simulink model "MyPCImages"  (Simulink 7.5)
settings: Solver=FixedStepDiscrete  StartTime=0.0  StopTime=d_data(end,1)  FixedStep=apSampleTime  RelTol=1e-3
InitFcn:
  | replayFlight
values from neighbouring files (symbols this model uses):
  apSampleTime = 0.01    [demoz2SlugsV5.m]
  D = y    [BarOrthog.m]
  R0 = single(Euler2DCMdeg( PHI_IC, THETA_IC, PSI_IC ))    [demoz2SlugsV5.m]
undefined symbols (not defined in the file or in its folder): accBiasRateLimit, accelXCutTemp, axTGain1, axTGain2, axTMean1, axTMean2, barAdjust, baroCutoff, baroCutTemp, baroOffset, baroScale, barTGain1, barTGain2, barTMean1, barTMean2, baseHeight, baseTemp, cubeAccelGain, cubeGyroGain, gaind, GS_location, gyroBiasRateLimit, Init_onlyOnce, Init_Reset, ISA_rho0, lapseRate, lowRateSensorCutoff, magMeanTemp, magOffset, magScale, magTempK, mainSensorCutoff, maxDynPressure, param_acc, param_mag, pitAdjust, pitCutTemp, pitotOffset, pitotScale, pitTGain1, pitTGain2, pitTMean1, pitTMean2, polesd, powerOffset, powerScale, pressureSensorCutoff, T, tempOffset, tempScale, vzCutoff, xCutoff, yCutoff, zCutoff, zerosd
libraries: simulink x11, aerolibconvert2 x9, SLUGS_Library x6, aerolibutil x3, dspmtrx3 x3, dsPICdrivers x1
(part 1 of 4)
Description:
  | Rodrigues' formula for rotations, eq'n (12) of
  | Park, Chung, 'Geometric Integration on Euclidean
  | Group with Application to Articulated Multibody Systems', 2005
settings Model: Creator=Administrator  LastModifiedBy=Robert
settings OptimizationCC: InitFltsAndDblsToZero=on
settings DebuggingCC: SaveWithParameterizedLinksMsg=none  StrictBusMsg=Warning
settings GRTTargetCC: TargetFcnLib=ansi_tfl_tmw.mat

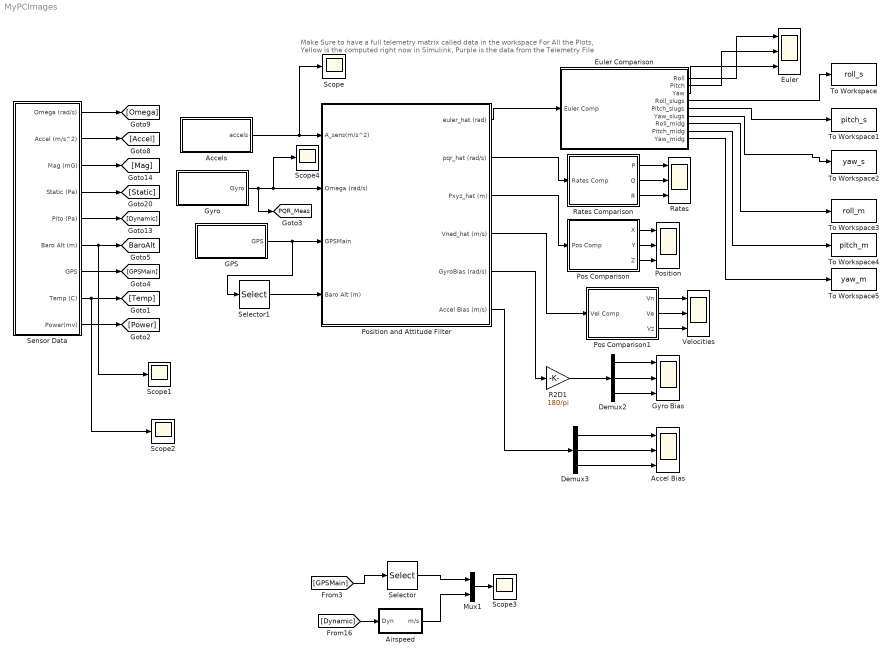
== system MyPCImages ==
  note: Make Sure to have a full telemetry matrix
      | called data in the workspace
      |
      | For All the Plots, Yellow is the computed right now in Simulink,
      |  Purple is the data from the Telemetry File
  Accel Bias : Scope  NumInputPorts=3
      settings: YMin=-0.05~-0.001~-1.73472e-018  YMax=0~0.0065~0.055  SaveName=ScopeData5
  Accels : Subsystem
  Airspeed : Subsystem
  Demux2 : Demux  Outputs=3
  Demux3 : Demux  Outputs=3
  Euler : Scope  NumInputPorts=3
      settings: YMin=-35~-7.5~0  YMax=10~10~400  SaveName=ScopeData15
  Euler Comparison : Subsystem
  GPS : Subsystem
  Gyro : Subsystem
  Gyro Bias : Scope  NumInputPorts=3
      settings: YMin=-0.1~5.55112e-017~-1  YMax=1~1.3~0.75  SaveName=ScopeData4
  Mux1 : Mux  Inputs=2
  Pos Comparison : Subsystem
  Pos Comparison1 : Subsystem
  Position : Scope  NumInputPorts=3
      settings: YMin=0~0~0  YMax=1.3e+006~2.25e+006~550000  SaveName=ScopeData2
  Position and Attitude Filter : Subsystem
  R2D1 : Gain  Gain=180/pi  ParameterDataType=sfix(16)  ParameterScaling=2^0  OutDataType=sfix(16)  OutScaling=2^0
  Rates : Scope  NumInputPorts=3
      settings: YMin=-150~-40~-70  YMax=150~80~40
  Rates Comparison : Subsystem
  Scope{,1..4} (5 alike) : Scope
      Scope settings: YMin=-22.5  YMax=15  SaveName=ScopeData10
      Scope1 settings: YMin=180  YMax=330  SaveName=ScopeData11
      Scope2 settings: TimeRange=300  YMin=-1200  YMax=400  SaveName=ScopeData6
      Scope3 settings: YMin=0  YMax=22.5  SaveName=ScopeData7
      Scope4 settings: YMin=-22.5  YMax=15
  Selector : Selector  InputPortWidth=5  IndexOptions=Index vector (dialog)  Indices=5  OutputSizes=1
  Selector1 : Selector  InputPortWidth=5  IndexOptions=Index vector (dialog)  Indices=3  OutputSizes=1
  Sensor Data : Subsystem
  To Workspace : ToWorkspace  VariableName=roll_s  SampleTime=-1  SaveFormat=Structure
  To Workspace1 : ToWorkspace  VariableName=pitch_s  SampleTime=-1  SaveFormat=Structure
  To Workspace2 : ToWorkspace  VariableName=yaw_s  SampleTime=-1  SaveFormat=Structure
  To Workspace3 : ToWorkspace  VariableName=roll_m  SampleTime=-1  SaveFormat=Structure
  To Workspace4 : ToWorkspace  VariableName=pitch_m  SampleTime=-1  SaveFormat=Structure
  To Workspace5 : ToWorkspace  VariableName=yaw_m  SampleTime=-1  SaveFormat=Structure
  Velocities : Scope  NumInputPorts=3
      settings: YMin=-25~-20~-15  YMax=25~25~17.5  SaveName=ScopeData3
  tag scope: BaroAlt=global, PQR_Meas=global
  wires:
  Accels/1(accels) -> Scope/1, Position and Attitude Filter/1(A_sens(m/s^2))
  GPS/1(GPS) -> Position and Attitude Filter/3(GPSMain), Selector1/1
  Sensor Data/2(Accel (m/s^2)) -> [Accel]
  Sensor Data/1(Omega (rad/s)) -> [Omega]
  Sensor Data/3(Mag (mG)) -> [Mag]
  Sensor Data/4(Static (Pa)) -> [Static]
  Sensor Data/5(Pito (Pa)) -> [Dynamic]
  Sensor Data/6(Baro Alt (m)) -> [BaroAlt], Scope1/1
  Sensor Data/7(GPS) -> [GPSMain]
  Sensor Data/8(Temp (C)) -> [Temp], Scope2/1
  Sensor Data/9(Power(mv)) -> [Power]
  Position and Attitude Filter/1(euler_hat (rad)) -> Euler Comparison/1(Euler Comp)
  Rates Comparison/1(P) -> Rates/1
  Rates Comparison/2(Q) -> Rates/2
  Rates Comparison/3(R) -> Rates/3
  Pos Comparison/3(Z) -> Position/3
  Position and Attitude Filter/3(Pxyz_hat (m)) -> Pos Comparison/1(Pos Comp)
  Pos Comparison/1(X) -> Position/1
  Pos Comparison/2(Y) -> Position/2
  Position and Attitude Filter/4(Vned_hat (m/s)) -> Pos Comparison1/1(Vel Comp)
  Demux2/3 -> Gyro Bias/3
  Demux2/2 -> Gyro Bias/2
  Demux2/1 -> Gyro Bias/1
  Position and Attitude Filter/5(GyroBias (rad/s)) -> R2D1/1
  Demux3/3 -> Accel Bias/3
  Demux3/2 -> Accel Bias/2
  Position and Attitude Filter/6(Accel Bias (m/s)) -> Demux3/1
  Demux3/1 -> Accel Bias/1
  Position and Attitude Filter/2(pqr_hat (rad/s)) -> Rates Comparison/1(Rates Comp)
  Pos Comparison1/1(Vn) -> Velocities/1
  Pos Comparison1/2(Ve) -> Velocities/2
  Pos Comparison1/3(Vz) -> Velocities/3
  R2D1/1 -> Demux2/1
  Gyro/1(Gyro) -> Position and Attitude Filter/2(Omega (rad/s)), Scope4/1, [PQR_Meas]
  Selector1/1 -> Position and Attitude Filter/4(Baro Alt (m))
  [Dynamic] -> Airspeed/1(Dyn)
  [GPSMain] -> Selector/1
  Selector/1 -> Mux1/1
  Airspeed/1(m/s) -> Mux1/2
  Mux1/1 -> Scope3/1
  Euler Comparison/1(Roll) -> Euler/1
  Euler Comparison/2(Pitch) -> Euler/2
  Euler Comparison/3(Yaw) -> Euler/3
  Euler Comparison/4(Roll_slugs) -> To Workspace/1
  Euler Comparison/5(Pitch_slugs) -> To Workspace1/1
  Euler Comparison/6(Yaw_slugs) -> To Workspace2/1
  Euler Comparison/7(Roll_midg) -> To Workspace3/1
  Euler Comparison/8(Pitch_midg) -> To Workspace4/1
  Euler Comparison/9(Yaw_midg) -> To Workspace5/1

== system MyPCImages/Accels ==
  Data Type Conversion : DataTypeConversion  OutDataTypeMode=single  OutDataType=sfix(16)  OutScaling=2^0  OutDataTypeStr=single
  Mux : Mux  Inputs=3
  p : FromWorkspace  VariableName=[d_data(:,1) d_data(:,5)]  SampleTime=0.01  OutputAfterFinalValue=Setting to zero
  p1 : FromWorkspace  VariableName=[d_data(:,1) d_data(:,6)]  SampleTime=0.01  OutputAfterFinalValue=Setting to zero
  p2 : FromWorkspace  VariableName=[d_data(:,1) d_data(:,7)]  SampleTime=0.01  OutputAfterFinalValue=Setting to zero
  accels : Outport  OutDataType=sfix(16)  OutScaling=2^0
  wires:
  Mux/1 -> Data Type Conversion/1
  p2/1 -> Mux/3
  p1/1 -> Mux/2
  p/1 -> Mux/1
  Data Type Conversion/1 -> accels/1

== system MyPCImages/Airspeed ==
  Dyn : Inport  OutDataType=sfix(16)  OutScaling=2^0
  Gain : Gain  Gain=2/ISA_rho0  ParameterDataType=sfix(16)  ParameterScaling=2^0  OutDataType=sfix(16)  OutScaling=2^0
  Math Function : Math  Operator=sqrt  OutDataType=sfix(16)  OutScaling=2^0  SaturateOnIntegerOverflow=on
  "[0.001  2000]" : Saturate  UpperLimit=2000  LowerLimit=0.001
  m/s : Outport  OutDataType=sfix(16)  OutScaling=2^0
  wires:
  "[0.001  2000]"/1 -> Math Function/1
  Math Function/1 -> m/s/1
  Dyn/1 -> Gain/1
  Gain/1 -> "[0.001  2000]"/1

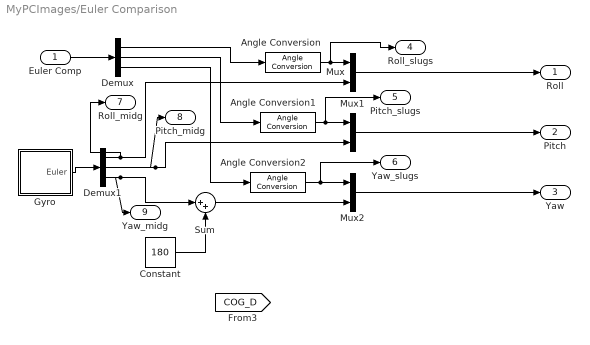
== system MyPCImages/Euler Comparison ==
  Euler Comp : Inport  OutDataType=sfix(16)  OutScaling=2^0
  Angle Conversion : aerolibconvert2/Angle Conversion  SystemSampleTime=-1  IU=rad  OU=deg
  Angle Conversion1 : aerolibconvert2/Angle Conversion  SystemSampleTime=-1  IU=rad  OU=deg
  Angle Conversion2 : aerolibconvert2/Angle Conversion  SystemSampleTime=-1  IU=rad  OU=deg
  Constant : Constant  Value=180  OutDataTypeMode=single  OutDataType=sfix(16)  OutScaling=2^0  OutDataTypeStr=single
  Demux : Demux  Outputs=3
  Demux1 : Demux  Outputs=3
  Gyro : Subsystem
  Mux : Mux  Inputs=2
  Mux1 : Mux  Inputs=2
  Mux2 : Mux  Inputs=2
  Sum : Sum  Inputs=|++  OutDataType=sfix(16)  OutScaling=2^0
  Roll : Outport  OutDataType=sfix(16)  OutScaling=2^0
  Pitch : Outport  Port=2  OutDataType=sfix(16)  OutScaling=2^0
  Yaw : Outport  Port=3  OutDataType=sfix(16)  OutScaling=2^0
  Roll_slugs : Outport  Port=4  OutDataType=sfix(16)  OutScaling=2^0
  Pitch_slugs : Outport  Port=5  OutDataType=sfix(16)  OutScaling=2^0
  Yaw_slugs : Outport  Port=6  OutDataType=sfix(16)  OutScaling=2^0
  Roll_midg : Outport  Port=7  OutDataType=sfix(16)  OutScaling=2^0
  Pitch_midg : Outport  Port=8  OutDataType=sfix(16)  OutScaling=2^0
  Yaw_midg : Outport  Port=9  OutDataType=sfix(16)  OutScaling=2^0
  wires:
  Mux/1 -> Roll/1
  Mux1/1 -> Pitch/1
  Mux2/1 -> Yaw/1
  Euler Comp/1 -> Demux/1
  Demux/1 -> Angle Conversion/1
  Demux/2 -> Angle Conversion1/1
  Demux/3 -> Angle Conversion2/1
  Gyro/1(Euler) -> Demux1/1
  Demux1/1 -> Mux/2, Roll_midg/1
  Demux1/2 -> Mux1/2, Pitch_midg/1
  Angle Conversion/1 -> Mux/1, Roll_slugs/1
  Angle Conversion1/1 -> Mux1/1, Pitch_slugs/1
  Angle Conversion2/1 -> Mux2/1, Yaw_slugs/1
  Sum/1 -> Mux2/2
  Demux1/3 -> Sum/1, Yaw_midg/1
  Constant/1 -> Sum/2

== system MyPCImages/GPS ==
  Data Type Conversion : DataTypeConversion  OutDataTypeMode=single  OutDataType=sfix(16)  OutScaling=2^0  OutDataTypeStr=single
  Mux : Mux  Inputs=5
  p : FromWorkspace  VariableName=[d_data(:,1) d_data(:,8)]  SampleTime=0.01  OutputAfterFinalValue=Setting to zero
  p1 : FromWorkspace  VariableName=[d_data(:,1) d_data(:,9)]  SampleTime=0.01  OutputAfterFinalValue=Setting to zero
  p2 : FromWorkspace  VariableName=[d_data(:,1) d_data(:,10)]  SampleTime=0.01  OutputAfterFinalValue=Setting to zero
  p3 : FromWorkspace  VariableName=[d_data(:,1) d_data(:,11)]  SampleTime=0.01  OutputAfterFinalValue=Setting to zero
  p4 : FromWorkspace  VariableName=[d_data(:,1) d_data(:,12)]  SampleTime=0.01  OutputAfterFinalValue=Setting to zero
  GPS : Outport  OutDataType=sfix(16)  OutScaling=2^0
  wires:
  p/1 -> Mux/1
  p1/1 -> Mux/2
  p2/1 -> Mux/3
  Mux/1 -> Data Type Conversion/1
  p3/1 -> Mux/4
  p4/1 -> Mux/5
  Data Type Conversion/1 -> GPS/1

== system MyPCImages/Gyro ==
  Data Type Conversion : DataTypeConversion  OutDataTypeMode=single  OutDataType=sfix(16)  OutScaling=2^0  OutDataTypeStr=single
  Mux : Mux  Inputs=3
  p : FromWorkspace  VariableName=[d_data(:,1) d_data(:,2)]  SampleTime=0.01  OutputAfterFinalValue=Setting to zero
  p1 : FromWorkspace  VariableName=[d_data(:,1) d_data(:,3)]  SampleTime=0.01  OutputAfterFinalValue=Setting to zero
  p2 : FromWorkspace  VariableName=[d_data(:,1) d_data(:,4)]  SampleTime=0.01  OutputAfterFinalValue=Setting to zero
  Gyro : Outport  OutDataType=sfix(16)  OutScaling=2^0
  wires:
  p/1 -> Mux/1
  p1/1 -> Mux/2
  p2/1 -> Mux/3
  Mux/1 -> Data Type Conversion/1
  Data Type Conversion/1 -> Gyro/1

== system MyPCImages/Pos Comparison ==
  Pos Comp : Inport  OutDataType=sfix(16)  OutScaling=2^0
  Demux : Demux  Outputs=3
  Demux1 : Demux  Outputs=3
  Mux : Mux  Inputs=2
  Mux1 : Mux  Inputs=2
  Mux2 : Mux  Inputs=2
  X : Outport  OutDataType=sfix(16)  OutScaling=2^0
  Y : Outport  Port=2  OutDataType=sfix(16)  OutScaling=2^0
  Z : Outport  Port=3  OutDataType=sfix(16)  OutScaling=2^0
  wires:
  Mux/1 -> X/1
  Mux1/1 -> Y/1
  Mux2/1 -> Z/1
  Pos Comp/1 -> Demux/1
  Demux/1 -> Mux/1
  Demux/2 -> Mux1/1
  Demux/3 -> Mux2/1
  [GPS_XYD] -> Demux1/1
  Demux1/1 -> Mux/2
  Demux1/2 -> Mux1/2
  Demux1/3 -> Mux2/2

== system MyPCImages/Pos Comparison1 ==
  Vel Comp : Inport  OutDataType=sfix(16)  OutScaling=2^0
  Demux : Demux  Outputs=3
  Mux : Mux  Inputs=2
  Mux1 : Mux  Inputs=2
  Mux2 : Mux  Inputs=2
  Vn : Outport  OutDataType=sfix(16)  OutScaling=2^0
  Ve : Outport  Port=2  OutDataType=sfix(16)  OutScaling=2^0
  Vz : Outport  Port=3  OutDataType=sfix(16)  OutScaling=2^0
  wires:
  ? -> Mux2/2
  [Veast] -> Mux1/2
  [Vnorth] -> Mux/2
  Demux/3 -> Mux2/1
  Demux/2 -> Mux1/1
  Demux/1 -> Mux/1
  Vel Comp/1 -> Demux/1
  Mux2/1 -> Vz/1
  Mux1/1 -> Ve/1
  Mux/1 -> Vn/1

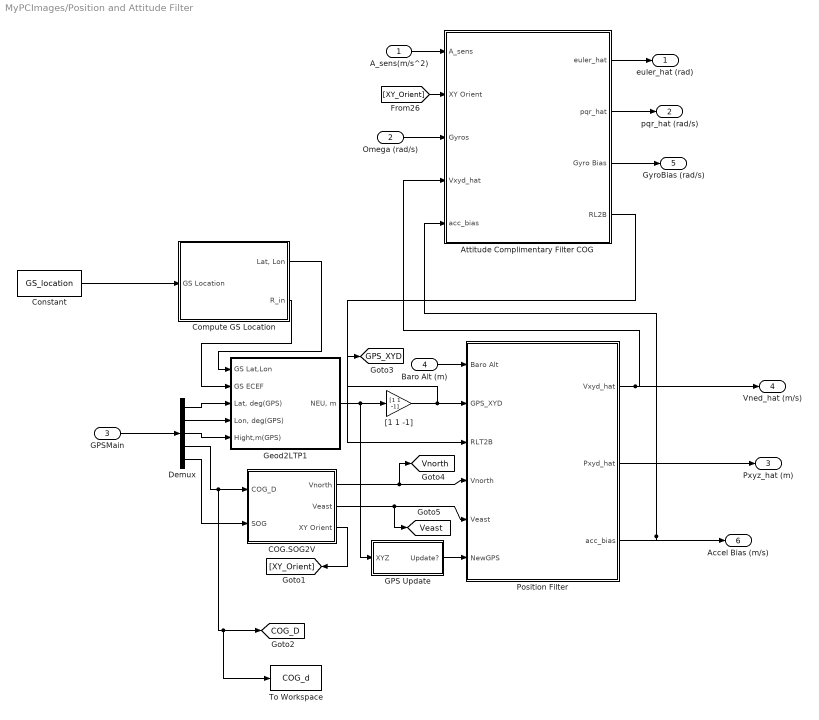
== system MyPCImages/Position and Attitude Filter ==
  A_sens(m/s^2) : Inport  OutDataType=sfix(16)  OutScaling=2^0
  Omega (rad/s) : Inport  Port=2  OutDataType=sfix(16)  OutScaling=2^0
  GPSMain : Inport  Port=3  OutDataType=sfix(16)  OutScaling=2^0
  Baro Alt (m) : Inport  Port=4  OutDataType=sfix(16)  OutScaling=2^0
  Attitude Complimentary Filter COG : Subsystem
  COG.SOG2V : Subsystem
  Compute GS Location : Subsystem
  Constant : Constant  Value=GS_location  OutDataTypeMode=single  OutDataType=sfix(16)  OutScaling=2^0  OutDataTypeStr=single
  Demux : Demux  Outputs=5
  GPS Update : Subsystem  mask{T=0.01}
      mask prompts: T "Sample Time"
  Geod2LTP1 : Subsystem
      mask Description:
      | This block provides transformation of the Geodetic coordinates
      | to the LTP coorinate system. The block uses two consecutive transformations
      | (Geodetic -> ECEF ->LTP).
      | Geodetic coordinates of the LTP origin should also be predetermined.
      mask Help: Oops!
      mask Display: plot(0,0,100,100,[45,40,35,40,40],[85,95,85,95,40],[85,95,85,95,40],[35,40,45,40,40],[60,40,10,20,10,14],[70,40,10,13,10,20],[56,45],[70,70],[60,60],[50,60],[60,60],[30,40],[50,60],[20,20],[30,40],[20,20],[45,55],[35,25],[75,65],[35,25])
  Position Filter : Subsystem
  To Workspace : ToWorkspace  VariableName=COG_d  SampleTime=-1  SaveFormat=Structure
  "[1 1 -1]" : Gain  Gain=[1 1 -1]  ParameterDataType=sfix(16)  ParameterScaling=2^0  OutDataType=sfix(16)  OutScaling=2^0
  euler_hat (rad) : Outport  OutDataType=sfix(16)  OutScaling=2^0
  pqr_hat (rad/s) : Outport  Port=2  OutDataType=sfix(16)  OutScaling=2^0
  Pxyz_hat (m) : Outport  Port=3  OutDataType=sfix(16)  OutScaling=2^0
  Vned_hat (m/s) : Outport  Port=4  OutDataType=sfix(16)  OutScaling=2^0
  GyroBias (rad/s) : Outport  Port=5  OutDataType=sfix(16)  OutScaling=2^0
  Accel Bias (m/s) : Outport  Port=6  OutDataType=sfix(16)  OutScaling=2^0
  tag scope: COG_D=global, GPS_XYD=global, Veast=global, Vnorth=global
  wires:
  COG.SOG2V/3(XY Orient) -> [XY_Orient]
  COG.SOG2V/2(Veast) -> Position Filter/5(Veast), [Veast]
  COG.SOG2V/1(Vnorth) -> Position Filter/4(Vnorth), [Vnorth]
  Demux/5 -> COG.SOG2V/2(SOG)
  Demux/4 -> COG.SOG2V/1(COG_D), [COG_D], To Workspace/1
  Baro Alt (m)/1 -> Position Filter/1(Baro Alt)
  [XY_Orient] -> Attitude Complimentary Filter COG/2(XY Orient)
  "[1 1 -1]"/1 -> Position Filter/2(GPS_XYD), [GPS_XYD]
  Omega (rad/s)/1 -> Attitude Complimentary Filter COG/3(Gyros)
  A_sens(m/s^2)/1 -> Attitude Complimentary Filter COG/1(A_sens)
  GPS Update/1(Update?) -> Position Filter/6(NewGPS)
  Compute GS Location/1("Lat, Lon") -> Geod2LTP1/1(GS Lat,Lon)
  Compute GS Location/2(R_in) -> Geod2LTP1/2(GS ECEF)
  Demux/3 -> Geod2LTP1/5(Hight,m(GPS))
  Demux/2 -> Geod2LTP1/4("Lon, deg(GPS)")
  Demux/1 -> Geod2LTP1/3("Lat, deg(GPS)")
  Constant/1 -> Compute GS Location/1(GS Location)
  GPSMain/1 -> Demux/1
  Attitude Complimentary Filter COG/3(Gyro Bias) -> GyroBias (rad/s)/1
  Attitude Complimentary Filter COG/2(pqr_hat) -> pqr_hat (rad/s)/1
  Attitude Complimentary Filter COG/1(euler_hat) -> euler_hat (rad)/1
  Attitude Complimentary Filter COG/4(RL2B) -> Position Filter/3(RLT2B)
  Geod2LTP1/1("NEU, m") -> "[1 1 -1]"/1, GPS Update/1(XYZ)
  Position Filter/3(acc_bias) -> Attitude Complimentary Filter COG/5(acc_bias), Accel Bias (m/s)/1
  Position Filter/2(Pxyd_hat) -> Pxyz_hat (m)/1
  Position Filter/1(Vxyd_hat) -> Attitude Complimentary Filter COG/4(Vxyd_hat), Vned_hat (m/s)/1

== system MyPCImages/Rates Comparison ==
  Rates Comp : Inport  OutDataType=sfix(16)  OutScaling=2^0
  Angle Conversion : aerolibconvert2/Angle Conversion  SystemSampleTime=-1  IU=rad  OU=deg
  Angle Conversion1 : aerolibconvert2/Angle Conversion  SystemSampleTime=-1  IU=rad  OU=deg
  Angle Conversion2 : aerolibconvert2/Angle Conversion  SystemSampleTime=-1  IU=rad  OU=deg
  Demux : Demux  Outputs=3
  Demux1 : Demux  Outputs=3
  Mux : Mux  Inputs=2
  Mux1 : Mux  Inputs=2
  Mux2 : Mux  Inputs=2
  P : Outport  OutDataType=sfix(16)  OutScaling=2^0
  Q : Outport  Port=2  OutDataType=sfix(16)  OutScaling=2^0
  R : Outport  Port=3  OutDataType=sfix(16)  OutScaling=2^0
  wires:
  Angle Conversion2/1 -> R/1
  Angle Conversion1/1 -> Q/1
  Angle Conversion/1 -> P/1
  Demux1/3 -> Mux2/2
  Demux1/2 -> Mux1/2
  Demux1/1 -> Mux/2
  [PQR_Meas] -> Demux1/1
  Demux/3 -> Mux2/1
  Demux/2 -> Mux1/1
  Demux/1 -> Mux/1
  Rates Comp/1 -> Demux/1
  Mux2/1 -> Angle Conversion2/1
  Mux1/1 -> Angle Conversion1/1
  Mux/1 -> Angle Conversion/1

== system MyPCImages/Sensor Data ==
  Sensor Suite : Subsystem
  Omega (rad/s) : Outport  OutDataType=sfix(16)  OutScaling=2^0
  Accel (m/s^2) : Outport  Port=2  OutDataType=sfix(16)  OutScaling=2^0
  Mag (mG) : Outport  Port=3  OutDataType=sfix(16)  OutScaling=2^0
  Static (Pa) : Outport  Port=4  OutDataType=sfix(16)  OutScaling=2^0
  Pito (Pa) : Outport  Port=5  OutDataType=sfix(16)  OutScaling=2^0
  Baro Alt (m) : Outport  Port=6  OutDataType=sfix(16)  OutScaling=2^0
  GPS : Outport  Port=7  OutDataType=sfix(16)  OutScaling=2^0
  Temp (C) : Outport  Port=8  OutDataType=sfix(16)  OutScaling=2^0
  Power(mv) : Outport  Port=9  OutDataType=sfix(16)  OutScaling=2^0
  wires:
  Sensor Suite/7(GPS) -> GPS/1
  Sensor Suite/6(Baro Alt (m)) -> Baro Alt (m)/1
  Sensor Suite/5(Pitot (Pa)) -> Pito (Pa)/1
  Sensor Suite/4(Static (Pa)) -> Static (Pa)/1
  Sensor Suite/3(Mag (normalized)) -> Mag (mG)/1
  Sensor Suite/2(Accel (m/s^2)) -> Accel (m/s^2)/1
  Sensor Suite/1(Omega (rad/s)) -> Omega (rad/s)/1
  Sensor Suite/8(Temp(C)) -> Temp (C)/1
  Sensor Suite/9(Power) -> Power(mv)/1

== system MyPCImages/Euler Comparison/Gyro ==
  Data Type Conversion : DataTypeConversion  OutDataTypeMode=single  OutDataType=sfix(16)  OutScaling=2^0  OutDataTypeStr=single
  Mux : Mux  Inputs=3
  p : FromWorkspace  VariableName=[d_data(:,1) d_data(:,13)]  SampleTime=0.01  OutputAfterFinalValue=Setting to zero
  p1 : FromWorkspace  VariableName=[d_data(:,1) d_data(:,14)]  SampleTime=0.01  OutputAfterFinalValue=Setting to zero
  p2 : FromWorkspace  VariableName=[d_data(:,1) d_data(:,15)]  SampleTime=0.01  OutputAfterFinalValue=Setting to zero
  Euler : Outport  OutDataType=sfix(16)  OutScaling=2^0
  wires:
  p/1 -> Mux/1
  p1/1 -> Mux/2
  p2/1 -> Mux/3
  Mux/1 -> Data Type Conversion/1
  Data Type Conversion/1 -> Euler/1

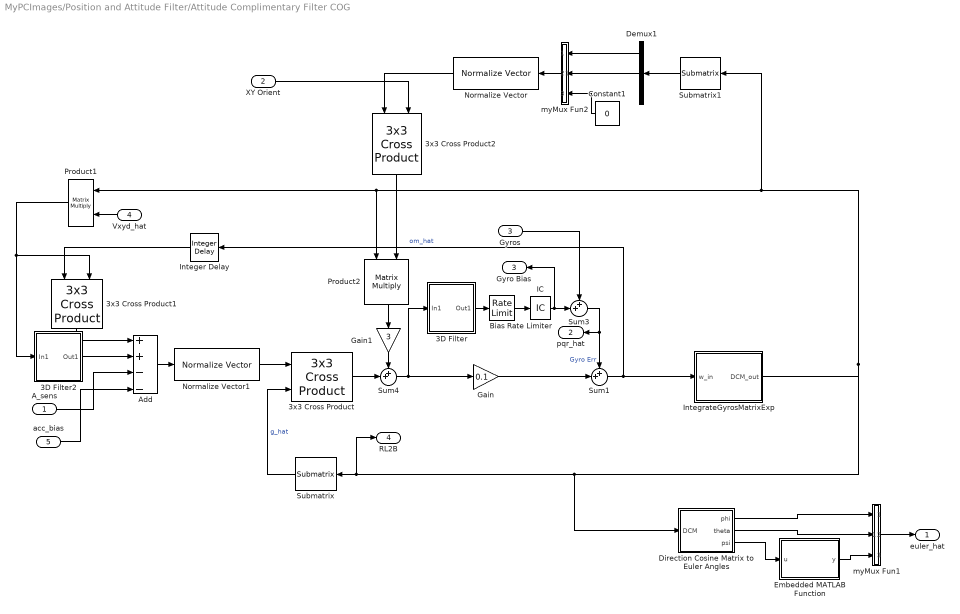
== system MyPCImages/Position and Attitude Filter/Attitude Complimentary Filter COG ==
  A_sens : Inport  PortDimensions=3  OutDataType=sfix(16)  OutScaling=2^0
  XY Orient : Inport  Port=2  DataType=single  OutDataType=sfix(16)  OutScaling=2^0  OutDataTypeStr=single
  Gyros : Inport  Port=3  PortDimensions=3  OutDataType=sfix(16)  OutScaling=2^0
  Vxyd_hat : Inport  Port=4  PortDimensions=3  OutDataType=sfix(16)  OutScaling=2^0
  acc_bias : Inport  Port=5  PortDimensions=3  OutDataType=sfix(16)  OutScaling=2^0
  3D Filter : Subsystem  AncestorBlock=SLUGS_Library/Singnal Routing & Conditioning/3D Filter  RTWFcnName=TustinFilter3D  mask{zval=[], pval=[0], kval=1, TSample=0.01}
      mask prompts: zval "Zeros"; pval "Poles"; kval "Gains"; TSample "Sample Time"
      settings: RTWFcnNameOpts=User specified  RTWFileNameOpts=Use function name
      mask Display:
      | droots(zval,pval,kval)
      | port_label('input',1,'3D')
  3D Filter2 : Subsystem  AncestorBlock=SLUGS_Library/Singnal Routing & Conditioning/3D Filter  RTWFcnName=TustinFilter3D  mask{zval=[0], pval=[-10], kval=10, TSample=0.01}
      mask prompts: zval "Zeros"; pval "Poles"; kval "Gains"; TSample "Sample Time"
      settings: RTWFcnNameOpts=User specified  RTWFileNameOpts=Use function name
      mask Display:
      | droots(zval,pval,kval)
      | port_label('input',1,'3D')
  3x3 Cross Product : aerolibutil/3x3 Cross Product  SystemSampleTime=-1
  3x3 Cross Product1 : aerolibutil/3x3 Cross Product  SystemSampleTime=-1
  3x3 Cross Product2 : aerolibutil/3x3 Cross Product  SystemSampleTime=-1
  Add : Sum  Inputs=++--  OutDataType=sfix(16)  OutScaling=2^-10
  Bias Rate Limiter : RateLimiter  RisingSlewLimit=gyroBiasRateLimit  FallingSlewLimit=-gyroBiasRateLimit  SampleTimeMode=inherited
  Constant1 : Constant  Value=0  OutDataTypeMode=single  OutDataType=sfix(16)  OutScaling=2^0  OutDataTypeStr=single
  Demux1 : Demux  Outputs=3
  Direction Cosine Matrix to Euler Angles : Subsystem  AncestorBlock=aerolibtransform2/Direction Cosine Matrix to Euler Angles  mask(DCM2Euler){}
      mask help: Determine an euler orientation (roll, pitch, yaw) from the 3-by-3 direction cosine matrix (DCM). The input DCM transforms vectors from geodetic earth or north-down-east (NED) axes to body axes.
      mask init:
      | aeroicon('aeroblk');
      mask Help: web(asbhelp('directioncosinematrixtoeulerangles'));
      mask Display:
      | port_label('output',1,'\phi','texmode','on')
      | port_label('output',2,'\theta','texmode','on')
      | port_label('output',3,'\psi','texmode','on')
      | port_label('input',1,'DCM_{be}','texmode','on')
  Embedded MATLAB Function : Stateflow chart  TreatAsAtomicUnit=on
  Gain : Gain  Gain=0.1  ParameterDataType=sfix(16)  ParameterScaling=2^0  OutDataType=sfix(16)  OutScaling=2^0
  Gain1 : Gain  Gain=3  ParameterDataType=sfix(16)  ParameterScaling=2^0  OutDataType=sfix(16)  OutScaling=2^0
  IC : InitialCondition  Value=0
  Integer Delay : simulink/Discrete/Integer Delay  vinit=0.0  samptime=-1  NumDelays=1
  IntegrateGyrosMatrixExp : Subsystem
  Normalize Vector : SLUGS_Library/Navigation/Normalize Vector  SystemSampleTime=-1
  Normalize Vector1 : SLUGS_Library/Navigation/Normalize Vector  SystemSampleTime=-1
  Product1 : Product  Multiplication=Matrix(*)  OutDataType=sfix(16)  OutScaling=2^0  RndMeth=Zero
  Product2 : Product  Multiplication=Matrix(*)  OutDataType=sfix(16)  OutScaling=2^0  RndMeth=Zero
  Submatrix : dspmtrx3/Submatrix  RowSpan=Range of rows  RowStartMode=First  RowStartIndex=1  RowEndMode=Last  RowEndIndex=1  ColSpan=One column  ColStartMode=Last  ColStartIndex=1  ColEndMode=Last  ColEndIndex=1
  Submatrix1 : dspmtrx3/Submatrix  RowSpan=One row  RowStartMode=First  RowStartIndex=1  RowEndMode=Last  RowEndIndex=1  ColSpan=All columns  ColStartMode=Last  ColStartIndex=1  ColEndMode=Last  ColEndIndex=1
  Sum1 : Sum  Inputs=++|  OutDataType=sfix(16)  OutScaling=2^0
  Sum3 : Sum  Inputs=++|  OutDataType=sfix(16)  OutScaling=2^0
  Sum4 : Sum  Inputs=++|  OutDataType=sfix(16)  OutScaling=2^0
  myMux Fun1 : Stateflow chart  TreatAsAtomicUnit=on
  myMux Fun2 : Stateflow chart  TreatAsAtomicUnit=on
  euler_hat : Outport  OutDataType=sfix(16)  OutScaling=2^0
  pqr_hat : Outport  Port=2  OutDataType=sfix(16)  OutScaling=2^0
  Gyro Bias : Outport  Port=3  OutDataType=sfix(16)  OutScaling=2^0
  RL2B : Outport  Port=4  OutDataType=sfix(16)  OutScaling=2^0
  wires:
  3x3 Cross Product2/1 -> Product2/2
  XY Orient/1 -> 3x3 Cross Product2/2
  Sum3/1 -> pqr_hat/1, Sum1/1  "Gyro Err"
  Gain/1 -> Sum1/2
  Gyros/1 -> Sum3/1
  3D Filter/1(Out1) -> Bias Rate Limiter/1
  Embedded MATLAB Function/1(y) -> myMux Fun1/3(u3)
  Direction Cosine Matrix to Euler Angles/2(theta) -> myMux Fun1/2(u2)
  Direction Cosine Matrix to Euler Angles/1(phi) -> myMux Fun1/1(u1)
  myMux Fun1/1(y) -> euler_hat/1
  Direction Cosine Matrix to Euler Angles/3(psi) -> Embedded MATLAB Function/1(u)
  Vxyd_hat/1 -> Product1/2
  Product1/1 -> 3x3 Cross Product1/2, 3D Filter2/1(In1)
  acc_bias/1 -> Add/4
  Add/1 -> Normalize Vector1/1
  3D Filter2/1(Out1) -> Add/2
  Integer Delay/1 -> 3x3 Cross Product1/1
  3x3 Cross Product/1 -> Sum4/2
  Normalize Vector1/1 -> 3x3 Cross Product/1
  A_sens/1 -> Add/3
  3x3 Cross Product1/1 -> Add/1
  Sum4/1 -> 3D Filter/1(In1), Gain/1
  Submatrix/1 -> 3x3 Cross Product/2  "g_hat"
  Sum1/1 -> Integer Delay/1, IntegrateGyrosMatrixExp/1(w_in)  "om_hat"
  Submatrix1/1 -> Demux1/1
  Demux1/1 -> myMux Fun2/1(u1)
  Demux1/2 -> myMux Fun2/2(u2)
  Constant1/1 -> myMux Fun2/3(u3)
  myMux Fun2/1(y) -> Normalize Vector/1
  Normalize Vector/1 -> 3x3 Cross Product2/1
  Gain1/1 -> Sum4/1
  Product2/1 -> Gain1/1
  Bias Rate Limiter/1 -> IC/1
  IC/1 -> Sum3/2, Gyro Bias/1
  IntegrateGyrosMatrixExp/1(DCM_out) -> RL2B/1, Submatrix/1, Direction Cosine Matrix to Euler Angles/1(DCM), Product1/1, Product2/1, Submatrix1/1

== system MyPCImages/Position and Attitude Filter/COG.SOG2V ==
  COG_D : Inport  OutDataType=sfix(16)  OutScaling=2^0
  SOG : Inport  Port=2  OutDataType=sfix(16)  OutScaling=2^0
  Angle Conversion : aerolibconvert2/Angle Conversion  SystemSampleTime=-1  IU=deg  OU=rad
  Constant : Constant  Value=0  OutDataTypeMode=single  OutDataType=sfix(16)  OutScaling=2^0  OutDataTypeStr=single
  Product : Product  OutDataType=sfix(16)  OutScaling=2^0  RndMeth=Zero
  Product1 : Product  OutDataType=sfix(16)  OutScaling=2^0  RndMeth=Zero
  Subsystem1 : SLUGS_Library/Subsystem5  SystemSampleTime=-1
  myMux Fun2 : Stateflow chart  TreatAsAtomicUnit=on
  Vnorth : Outport  OutDataType=sfix(16)  OutScaling=2^0
  Veast : Outport  Port=2  OutDataType=sfix(16)  OutScaling=2^0
  XY Orient : Outport  Port=3  OutDataType=sfix(16)  OutScaling=2^0
  wires:
  myMux Fun2/1(y) -> XY Orient/1
  Constant/1 -> myMux Fun2/3(u3)
  COG_D/1 -> Angle Conversion/1
  Subsystem1/2 -> myMux Fun2/1(u1), Product1/2
  Subsystem1/1 -> myMux Fun2/2(u2), Product/1
  Angle Conversion/1 -> Subsystem1/1
  SOG/1 -> Product/2, Product1/1
  Product/1 -> Veast/1
  Product1/1 -> Vnorth/1

== system MyPCImages/Position and Attitude Filter/Compute GS Location ==
  GS Location : Inport  OutDataType=sfix(16)  OutScaling=2^0
  Demux : Demux  Outputs=3
  Geod2ECEF1 : Subsystem  mask{Re=6378137, Rp=6356752.3142}
      mask prompts: Re "Enter equatorial radius, m"; Rp "Enter polar radius,m"
  Mux1 : Mux  Inputs=2
  Mux2 : Mux  Inputs=3
  "Lat, Lon" : Outport  OutDataType=sfix(16)  OutScaling=2^0
  R_in : Outport  Port=2  OutDataType=sfix(16)  OutScaling=2^0
  wires:
  Mux2/1 -> R_in/1  "R_in"
  Mux1/1 -> "Lat, Lon"/1
  GS Location/1 -> Demux/1
  Demux/3 -> Geod2ECEF1/3(lon,deg), Mux1/1
  Demux/2 -> Geod2ECEF1/2("lat, deg"), Mux1/2
  Demux/1 -> Geod2ECEF1/1("height, m")
  Geod2ECEF1/2("Ye, m ") -> Mux2/2
  Geod2ECEF1/1("Xe, m ") -> Mux2/1
  Geod2ECEF1/3("Ze, m ") -> Mux2/3

== system MyPCImages/Position and Attitude Filter/GPS Update ==
  XYZ : Inport  OutDataType=sfix(16)  OutScaling=2^0
  Data Type Conversion2 : DataTypeConversion  OutDataTypeMode=uint8  OutDataType=sfix(16)  OutScaling=2^0  OutDataTypeStr=uint8
  Demux : Demux  Outputs=3
  Detect Change : Subsystem
  Detect Change1 : Subsystem
  Detect Change2 : Subsystem
  Rate Transition : RateTransition  OutPortSampleTime=T
  Saturation1 : Saturate  UpperLimit=1  LowerLimit=0  SampleTime=T
  Sum : Sum  Inputs=3  OutDataType=sfix(16)  OutScaling=2^0
  Update? : Outport  OutDataType=sfix(16)  OutScaling=2^0
  wires:
  Data Type Conversion2/1 -> Update?/1
  Rate Transition/1 -> Demux/1
  Saturation1/1 -> Data Type Conversion2/1
  XYZ/1 -> Rate Transition/1
  Sum/1 -> Saturation1/1
  Detect Change2/1(change?) -> Sum/3
  Detect Change1/1(change?) -> Sum/2
  Detect Change/1(change?) -> Sum/1
  Demux/3 -> Detect Change2/1(Data)
  Demux/2 -> Detect Change1/1(Data)
  Demux/1 -> Detect Change/1(Data)

== system MyPCImages/Position and Attitude Filter/Geod2LTP1 ==
  GS Lat,Lon : Inport  OutDataType=sfix(16)  OutScaling=2^0
  GS ECEF : Inport  Port=2  OutDataType=sfix(16)  OutScaling=2^0
  "Lat, deg(GPS)" : Inport  Port=3  OutDataType=sfix(16)  OutScaling=2^0
  "Lon, deg(GPS)" : Inport  Port=4  OutDataType=sfix(16)  OutScaling=2^0
  Hight,m(GPS) : Inport  Port=5  OutDataType=sfix(16)  OutScaling=2^0
  ECEF2LTP (UEN) : Subsystem
      mask Display: plot(0,0,100,100,[45,40,35,40,40],[85,95,85,95,40],[85,95,85,95,40],[35,40,45,40,40],[60,40,10,20,10,14],[70,40,10,13,10,20],[56,45],[70,70],[60,60],[50,60],[60,60],[30,40],[50,60],[20,20],[30,40],[20,20],[45,55],[35,25],[75,65],[35,25])
  Geod2ECEF1 : Subsystem  mask{Re=6378137, Rp=6356752.3142}
      mask prompts: Re "Enter equatorial radius, m"; Rp "Enter polar radius,m"
  Mux : Mux  Inputs=3
  Reshape : Reshape  OutputDimensionality=Column vector (2-D)
  Reshape1 : Reshape
  Sum1 : Sum  Inputs=|+-  OutDataTypeMode=single  OutDataType=sfix(16)  OutScaling=2^0  OutDataTypeStr=single  SaturateOnIntegerOverflow=on
  UEN 2 NEU : Gain  Gain=[0 0 1;0 1 0;1 0 0]  Multiplication=Matrix(K*u)  ParameterDataType=sfix(16)  ParameterScaling=2^0  OutDataTypeMode=Specify via dialog  OutDataType=float('single')  OutDataTypeStr=float('single')  SaturateOnIntegerOverflow=on  ParamDataTypeStr=Inherit: Same as input
  "NEU, m" : Outport  OutDataType=sfix(16)  OutScaling=2^0
  wires:
  UEN 2 NEU/1 -> Reshape1/1
  Geod2ECEF1/3("Ze, m ") -> Mux/3
  Geod2ECEF1/1("Xe, m ") -> Mux/1
  Geod2ECEF1/2("Ye, m ") -> Mux/2
  "Lat, deg(GPS)"/1 -> Geod2ECEF1/2("lat, deg")
  "Lon, deg(GPS)"/1 -> Geod2ECEF1/3(lon,deg)
  GS Lat,Lon/1 -> ECEF2LTP (UEN)/2("Long, Lat")
  GS ECEF/1 -> Sum1/2
  ECEF2LTP (UEN)/1(Out) -> Reshape/1  "Moving Side"
  Hight,m(GPS)/1 -> Geod2ECEF1/1("height, m")
  Mux/1 -> Sum1/1  "r_mov"
  Sum1/1 -> ECEF2LTP (UEN)/1(ECEF coordinates)
  Reshape/1 -> UEN 2 NEU/1
  Reshape1/1 -> "NEU, m"/1

== system MyPCImages/Position and Attitude Filter/Position Filter ==
  Baro Alt : Inport  OutDataType=sfix(16)  OutScaling=2^0
  GPS_XYD : Inport  Port=2  OutDataType=sfix(16)  OutScaling=2^0
  RLT2B : Inport  Port=3  OutDataType=sfix(16)  OutScaling=2^0
  Vnorth : Inport  Port=4  OutDataType=sfix(16)  OutScaling=2^0
  Veast : Inport  Port=5  OutDataType=sfix(16)  OutScaling=2^0
  NewGPS : Inport  Port=6  OutDataType=sfix(16)  OutScaling=2^0
  BlendPosVel : Subsystem
  Vxyd_hat : Outport  OutDataType=sfix(16)  OutScaling=2^0
  Pxyd_hat : Outport  Port=2  OutDataType=sfix(16)  OutScaling=2^0
  acc_bias : Outport  Port=3  OutDataType=sfix(16)  OutScaling=2^0
  wires:
  GPS_XYD/1 -> BlendPosVel/1(GPS_NED)
  RLT2B/1 -> BlendPosVel/5(RLT2B)
  NewGPS/1 -> BlendPosVel/6(NewGPS)
  Vnorth/1 -> BlendPosVel/2(Vnorth)
  Veast/1 -> BlendPosVel/3(Veast)
  Baro Alt/1 -> BlendPosVel/4(BaroAlt)
  BlendPosVel/2(Pxyd_hat) -> Pxyd_hat/1
  BlendPosVel/1(Vxyd_hat) -> Vxyd_hat/1
  BlendPosVel/3(acc_bias) -> acc_bias/1

== system MyPCImages/Sensor Data/Sensor Suite ==
  Cube Signal Cond : Subsystem
  Demux : Demux  Outputs=[3 3 3 4]
  Demux1 : Demux
  If no HIL then Read all the Sensors : Subsystem
  Low Pass Filtering,Temperature Compensation and Calibration : Subsystem
  Scope : Scope
      settings: SaveName=ScopeData9
  Omega (rad/s) : Outport  OutDataType=sfix(16)  OutScaling=2^0
  Accel (m/s^2) : Outport  Port=2  OutDataType=sfix(16)  OutScaling=2^0
  Mag (normalized) : Outport  Port=3  OutDataType=sfix(16)  OutScaling=2^0
  Static (Pa) : Outport  Port=4  OutDataType=sfix(16)  OutScaling=2^0
  Pitot (Pa) : Outport  Port=5  OutDataType=sfix(16)  OutScaling=2^0
  Baro Alt (m) : Outport  Port=6  OutDataType=sfix(16)  OutScaling=2^0
  GPS : Outport  Port=7  OutDataType=sfix(16)  OutScaling=2^0
  Temp(C) : Outport  Port=8  OutDataType=sfix(16)  OutScaling=2^0
  Power : Outport  Port=9  OutDataType=sfix(16)  OutScaling=2^0
  wires:
  Cube Signal Cond/2(Accel (m/s^2)) -> Accel (m/s^2)/1, Scope/1
  Cube Signal Cond/1(Omega (rad/s)) -> Omega (rad/s)/1
  Demux/2 -> Cube Signal Cond/2(Accel Raw)  "Accel"
  Low Pass Filtering,Temperature Compensation and Calibration/4(Magnetometer (normalized)) -> Mag (normalized)/1
  Low Pass Filtering,Temperature Compensation and Calibration/3(Static (Pa)) -> Static (Pa)/1
  Low Pass Filtering,Temperature Compensation and Calibration/2(Pitot (Pa)) -> Pitot (Pa)/1
  Demux1/3 -> Low Pass Filtering,Temperature Compensation and Calibration/4(Power Raw)
  Demux/3 -> Low Pass Filtering,Temperature Compensation and Calibration/1(Magnetometers Raw)  "Magnetometers Raw"
  Demux1/4 -> Low Pass Filtering,Temperature Compensation and Calibration/5(Therm Raw)
  Demux1/2 -> Low Pass Filtering,Temperature Compensation and Calibration/3(Pitot raw)
  Demux1/1 -> Low Pass Filtering,Temperature Compensation and Calibration/2(Baro raw)
  Demux/4 -> Demux1/1  "Air Data"
  Demux/1 -> Cube Signal Cond/1(Gyro Raw)  "Gyro"
  Low Pass Filtering,Temperature Compensation and Calibration/1(Baro Alt (m)) -> Baro Alt (m)/1
  If no HIL then Read all the Sensors/1(Sensors) -> Demux/1
  If no HIL then Read all the Sensors/2(GPS) -> GPS/1
  Low Pass Filtering,Temperature Compensation and Calibration/5(Temp (0.1 C)) -> Temp(C)/1, Cube Signal Cond/3(Temp)
  Low Pass Filtering,Temperature Compensation and Calibration/6(Power (V)) -> Power/1

== system MyPCImages/Position and Attitude Filter/Attitude Complimentary Filter COG/3D Filter ==
  In1 : Inport  OutDataType=sfix(16)  OutScaling=2^0
  Data Type Conversion1 : DataTypeConversion  OutDataTypeMode=single  OutDataType=sfix(16)  OutScaling=2^0  OutDataTypeStr=single
  Data Type Conversion2 : DataTypeConversion  OutDataTypeMode=double  OutDataType=sfix(16)  OutScaling=2^0  OutDataTypeStr=double
  Demux : Demux  Outputs=3
  Filter1 : Subsystem  mask(DiscretizedZeroPole){Zeros=zval, Poles=pval, Gain=kval, AbsTol=auto, SampleTime=TSample, method=tustin, Wc=1}
      mask prompts: Zeros "Zeros (enter in s-main:)"; Poles "Poles (enter in s-domain:)"; Gain "Gain (enter in s-domain:)"; AbsTol "Absolute tolerance:"; SampleTime "Sample time:"; Wc "Critical Frequency (Hz):"
      mask help: Continuous mask uses c2d to transform parameters onto the Discrete Zero-Pole block inside.
      mask init:
      | st=SampleTime;
      | if length(st)>1
      |     st=SampleTime(1);
      | end
      | if(st>0)
      |     [zerosd,polesd,gaind] = sldiscutil('disczpk', {st,method,Wc,Zeros,Poles,Gain});
      | end	
      | s = get_param(gcb,'maskvalues');
      | zeross = s{1};
      | poless = s{2};
      | gainss = s{3};
      | %zerosc = eval(zeross);
      | %polesc = eval(poless);
      | %gainsc = eval(gainss);
      | sldiscutil('initzpkmask', st);
      | if(st==0)
      | set_param([gcb '/Zero Pole'], 'AbsoluteTolerance', AbsTol);
      | end
      mask StyleString: edit,edit,edit,edit,edit,popup(zoh|foh|tustin|prewarp|matched),edit
      mask CallbackString: |||||hidecrit|
      mask Display:
      | droots(zeross,poless,gainss)
      | text( 0.5, 1.0, method, 'verticalAlignment','top')
  Filter2 : Subsystem  mask(DiscretizedZeroPole){Zeros=zval, Poles=pval, Gain=kval, AbsTol=auto, SampleTime=TSample, method=tustin, Wc=1}
      mask prompts: Zeros "Zeros (enter in s-main:)"; Poles "Poles (enter in s-domain:)"; Gain "Gain (enter in s-domain:)"; AbsTol "Absolute tolerance:"; SampleTime "Sample time:"; Wc "Critical Frequency (Hz):"
      mask help: Continuous mask uses c2d to transform parameters onto the Discrete Zero-Pole block inside.
      mask init: same as MyPCImages/Position and Attitude Filter/Attitude Complimentary Filter COG/3D Filter/Filter1
      mask StyleString: edit,edit,edit,edit,edit,popup(zoh|foh|tustin|prewarp|matched),edit
      mask CallbackString: |||||hidecrit|
      mask Display:
      | droots(zeross,poless,gainss)
      | text( 0.5, 1.0, method, 'verticalAlignment','top')
  Filter3 : Subsystem  mask(DiscretizedZeroPole){Zeros=zval, Poles=pval, Gain=kval, AbsTol=auto, SampleTime=TSample, method=tustin, Wc=1}
      mask prompts: Zeros "Zeros (enter in s-main:)"; Poles "Poles (enter in s-domain:)"; Gain "Gain (enter in s-domain:)"; AbsTol "Absolute tolerance:"; SampleTime "Sample time:"; Wc "Critical Frequency (Hz):"
      mask help: Continuous mask uses c2d to transform parameters onto the Discrete Zero-Pole block inside.
      mask init: same as MyPCImages/Position and Attitude Filter/Attitude Complimentary Filter COG/3D Filter/Filter1
      mask StyleString: edit,edit,edit,edit,edit,popup(zoh|foh|tustin|prewarp|matched),edit
      mask CallbackString: |||||hidecrit|
      mask Display:
      | droots(zeross,poless,gainss)
      | text( 0.5, 1.0, method, 'verticalAlignment','top')
  myMux Fun1 : Stateflow chart  TreatAsAtomicUnit=on
  Out1 : Outport  OutDataType=sfix(16)  OutScaling=2^0
  wires:
  Data Type Conversion1/1 -> Out1/1
  Data Type Conversion2/1 -> Demux/1
  Demux/1 -> Filter1/1(In1)
  Demux/2 -> Filter2/1(In1)
  Demux/3 -> Filter3/1(In1)
  Filter1/1(Out1) -> myMux Fun1/1(u1)
  Filter2/1(Out1) -> myMux Fun1/2(u2)
  Filter3/1(Out1) -> myMux Fun1/3(u3)
  In1/1 -> Data Type Conversion2/1
  myMux Fun1/1(y) -> Data Type Conversion1/1

== system MyPCImages/Position and Attitude Filter/Attitude Complimentary Filter COG/3D Filter2 ==
  In1 : Inport  OutDataType=sfix(16)  OutScaling=2^0
  Data Type Conversion1 : DataTypeConversion  OutDataTypeMode=single  OutDataType=sfix(16)  OutScaling=2^0  OutDataTypeStr=single
  Data Type Conversion2 : DataTypeConversion  OutDataTypeMode=double  OutDataType=sfix(16)  OutScaling=2^0  OutDataTypeStr=double
  Demux : Demux  Outputs=3
  Filter1 : Subsystem  mask(DiscretizedZeroPole){Zeros=zval, Poles=pval, Gain=kval, AbsTol=auto, SampleTime=TSample, method=tustin, Wc=1}
      mask prompts: Zeros "Zeros (enter in s-main:)"; Poles "Poles (enter in s-domain:)"; Gain "Gain (enter in s-domain:)"; AbsTol "Absolute tolerance:"; SampleTime "Sample time:"; Wc "Critical Frequency (Hz):"
      mask help: Continuous mask uses c2d to transform parameters onto the Discrete Zero-Pole block inside.
      mask init: same as MyPCImages/Position and Attitude Filter/Attitude Complimentary Filter COG/3D Filter/Filter1
      mask StyleString: edit,edit,edit,edit,edit,popup(zoh|foh|tustin|prewarp|matched),edit
      mask CallbackString: |||||hidecrit|
      mask Display:
      | droots(zeross,poless,gainss)
      | text( 0.5, 1.0, method, 'verticalAlignment','top')
  Filter2 : Subsystem  mask(DiscretizedZeroPole){Zeros=zval, Poles=pval, Gain=kval, AbsTol=auto, SampleTime=TSample, method=tustin, Wc=1}
      mask prompts: Zeros "Zeros (enter in s-main:)"; Poles "Poles (enter in s-domain:)"; Gain "Gain (enter in s-domain:)"; AbsTol "Absolute tolerance:"; SampleTime "Sample time:"; Wc "Critical Frequency (Hz):"
      mask help: Continuous mask uses c2d to transform parameters onto the Discrete Zero-Pole block inside.
      mask init: same as MyPCImages/Position and Attitude Filter/Attitude Complimentary Filter COG/3D Filter/Filter1
      mask StyleString: edit,edit,edit,edit,edit,popup(zoh|foh|tustin|prewarp|matched),edit
      mask CallbackString: |||||hidecrit|
      mask Display:
      | droots(zeross,poless,gainss)
      | text( 0.5, 1.0, method, 'verticalAlignment','top')
  Filter3 : Subsystem  mask(DiscretizedZeroPole){Zeros=zval, Poles=pval, Gain=kval, AbsTol=auto, SampleTime=TSample, method=tustin, Wc=1}
      mask prompts: Zeros "Zeros (enter in s-main:)"; Poles "Poles (enter in s-domain:)"; Gain "Gain (enter in s-domain:)"; AbsTol "Absolute tolerance:"; SampleTime "Sample time:"; Wc "Critical Frequency (Hz):"
      mask help: Continuous mask uses c2d to transform parameters onto the Discrete Zero-Pole block inside.
      mask init: same as MyPCImages/Position and Attitude Filter/Attitude Complimentary Filter COG/3D Filter/Filter1
      mask StyleString: edit,edit,edit,edit,edit,popup(zoh|foh|tustin|prewarp|matched),edit
      mask CallbackString: |||||hidecrit|
      mask Display:
      | droots(zeross,poless,gainss)
      | text( 0.5, 1.0, method, 'verticalAlignment','top')
  myMux Fun1 : Stateflow chart  TreatAsAtomicUnit=on
  Out1 : Outport  OutDataType=sfix(16)  OutScaling=2^0
  wires:
  Data Type Conversion1/1 -> Out1/1
  Data Type Conversion2/1 -> Demux/1
  Demux/1 -> Filter1/1(In1)
  Demux/2 -> Filter2/1(In1)
  Demux/3 -> Filter3/1(In1)
  Filter1/1(Out1) -> myMux Fun1/1(u1)
  Filter2/1(Out1) -> myMux Fun1/2(u2)
  Filter3/1(Out1) -> myMux Fun1/3(u3)
  In1/1 -> Data Type Conversion2/1
  myMux Fun1/1(y) -> Data Type Conversion1/1

== system MyPCImages/Position and Attitude Filter/Attitude Complimentary Filter COG/Direction Cosine Matrix to Euler Angles ==
  DCM : Inport  PortDimensions=[3,3]  OutDataType=sfix(16)  OutScaling=2^0
  "Reshape 3x3 -> 9" : Reshape  OutputDimensions=[9, 1]
  Subsystem1 : SLUGS_Library/Subsystem4  SystemSampleTime=-1
  Subsystem2 : SLUGS_Library/Subsystem4  SystemSampleTime=-1
  Subsystem3 : SLUGS_Library/Subsystem6  SystemSampleTime=-1
  cos(phi)cos(theta) : Subsystem
  cos(psi)cos(theta) : Subsystem
  sin(phi)cos(theta) : Subsystem
  sin(psi)cos(theta) : Subsystem
  sin(theta) : Subsystem
  phi : Outport  PortDimensions=1  OutDataType=sfix(16)  OutScaling=2^0  InitialOutput=0
  theta : Outport  Port=2  PortDimensions=1  OutDataType=sfix(16)  OutScaling=2^0  InitialOutput=0
  psi : Outport  Port=3  PortDimensions=1  OutDataType=sfix(16)  OutScaling=2^0  InitialOutput=0
  wires:
  DCM/1 -> "Reshape 3x3 -> 9"/1
  "Reshape 3x3 -> 9"/1 -> sin(theta)/1(DCM), cos(phi)cos(theta)/1(DCM), sin(phi)cos(theta)/1(DCM), cos(psi)cos(theta)/1(DCM), sin(psi)cos(theta)/1(DCM)
  sin(theta)/1(sin(theta)) -> Subsystem3/1
  sin(phi)cos(theta)/1(sin(phi)cos(theta)) -> Subsystem2/1
  cos(phi)cos(theta)/1(cos(phi)cos(theta)) -> Subsystem2/2
  sin(psi)cos(theta)/1(sin(psi)cos(theta)) -> Subsystem1/1
  cos(psi)cos(theta)/1(cos(psi)cos(theta)) -> Subsystem1/2
  Subsystem2/1 -> phi/1  "phi"
  Subsystem3/1 -> theta/1  "theta"
  Subsystem1/1 -> psi/1  "psi"

== system MyPCImages/Position and Attitude Filter/Attitude Complimentary Filter COG/IntegrateGyrosMatrixExp ==
  note: Integration of DCM using the closed form version of the matrix exponential:
      | R_dot = -w x R
      | Solution:  R_{k+1} = Rexp() * R_k, where  = e^{-w x dt}.
      | Initialization:  seed R_k with R_0 = identity matrix
  w_in : Inport
  Angle Conversion : aerolibconvert2/Angle Conversion  SystemSampleTime=-1  IU=deg  OU=rad
  Data Type Conversion : DataTypeConversion  OutDataTypeMode=single  OutDataType=fixdt(1, 16)  OutScaling=2^0  OutDataTypeStr=single
  IC1 : InitialCondition  Value=R0
  Integer Delay : simulink/Discrete/Integer Delay  vinit=0.0  samptime=-1  NumDelays=1
  "Rexp, Rodrigues formula" : Subsystem
  Rk+1 = Rexp()*Rk : Product  Multiplication=Matrix(*)  OutDataTypeMode=double  OutDataType=sfix(16)  OutScaling=2^0  OutDataTypeStr=double  RndMeth=Zero
  DCM_out : Outport
  wires:
  w_in/1 -> Angle Conversion/1
  Data Type Conversion/1 -> DCM_out/1
  Angle Conversion/1 -> "Rexp, Rodrigues formula"/1(w)
  Rk+1 = Rexp()*Rk/1 -> Integer Delay/1  "RLT2B"
  IC1/1 -> Data Type Conversion/1, Rk+1 = Rexp()*Rk/2
  Integer Delay/1 -> IC1/1
  "Rexp, Rodrigues formula"/1(exp_w) -> Rk+1 = Rexp()*Rk/1

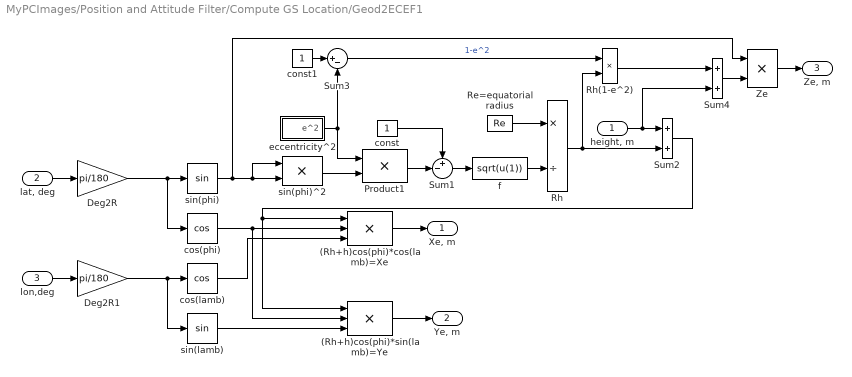
== system MyPCImages/Position and Attitude Filter/Compute GS Location/Geod2ECEF1 ==
  "height, m" : Inport  OutDataType=sfix(16)  OutScaling=2^0
  "lat, deg" : Inport  Port=2  OutDataType=sfix(16)  OutScaling=2^0
  lon,deg : Inport  Port=3  OutDataType=sfix(16)  OutScaling=2^0
  (Rh+h)cos(phi)*cos(lamb)=Xe : Product  Inputs=3  OutDataTypeMode=single  OutDataType=sfix(16)  OutScaling=2^0  OutDataTypeStr=single  SaturateOnIntegerOverflow=on  InputSameDT=on
  (Rh+h)cos(phi)*sin(lamb)=Ye : Product  Inputs=3  OutDataTypeMode=single  OutDataType=sfix(16)  OutScaling=2^0  OutDataTypeStr=single  SaturateOnIntegerOverflow=on  InputSameDT=on
  Deg2R : Gain  Gain=pi/180  ParameterDataType=sfix(16)  ParameterScaling=2^0  OutDataTypeMode=Specify via dialog  OutDataType=float('single')  OutDataTypeStr=float('single')  SaturateOnIntegerOverflow=on  ParamDataTypeStr=Inherit: Same as input
  Deg2R1 : Gain  Gain=pi/180  ParameterDataType=sfix(16)  ParameterScaling=2^0  OutDataTypeMode=Specify via dialog  OutDataType=float('single')  OutDataTypeStr=float('single')  SaturateOnIntegerOverflow=on  ParamDataTypeStr=Inherit: Same as input
  Product1 : Product  OutDataType=sfix(16)  OutScaling=2^0  SaturateOnIntegerOverflow=on  InputSameDT=on  OutDataTypeStr=Inherit: Same as first input
  Re=equatorial radius : Constant  Value=Re  OutDataTypeMode=single  OutDataType=sfix(16)  OutScaling=2^0  OutDataTypeStr=single
  Rh : Product  Inputs=*/  OutDataTypeMode=single  OutDataType=sfix(16)  OutScaling=2^0  OutDataTypeStr=single  SaturateOnIntegerOverflow=on  InputSameDT=on
  Rh(1-e^2) : Product  OutDataTypeMode=single  OutDataType=sfix(16)  OutScaling=2^0  OutDataTypeStr=single  SaturateOnIntegerOverflow=on  InputSameDT=on
  Sum1 : Sum  Inputs=+-|  OutDataType=sfix(16)  OutScaling=2^0  SaturateOnIntegerOverflow=on  InputSameDT=on  OutDataTypeStr=Inherit: Same as first input
  Sum2 : Sum  OutDataType=sfix(16)  OutScaling=2^0  SaturateOnIntegerOverflow=on  InputSameDT=on  OutDataTypeStr=Inherit: Same as first input
      settings: AttributesFormatString=Rh+h
  Sum3 : Sum  Inputs=|+-  OutDataType=sfix(16)  OutScaling=2^0  SaturateOnIntegerOverflow=on  InputSameDT=on  OutDataTypeStr=Inherit: Same as first input
  Sum4 : Sum  OutDataTypeMode=single  OutDataType=sfix(16)  OutScaling=2^0  OutDataTypeStr=single  SaturateOnIntegerOverflow=on  InputSameDT=on
      settings: AttributesFormatString=(1-e^2)Rh+h
  Ze : Product  OutDataTypeMode=single  OutDataType=sfix(16)  OutScaling=2^0  OutDataTypeStr=single  SaturateOnIntegerOverflow=on  InputSameDT=on
  const : Constant  OutDataTypeMode=single  OutDataType=sfix(16)  OutScaling=2^0  OutDataTypeStr=single
  const1 : Constant  OutDataTypeMode=single  OutDataType=sfix(16)  OutScaling=2^0  OutDataTypeStr=single
  cos(lamb) : Trigonometry  Operator=cos
  cos(phi) : Trigonometry  Operator=cos
  eccentricity^2 : Subsystem
  f : Fcn  Expr=sqrt(u(1))
  sin(lamb) : Trigonometry
  sin(phi) : Trigonometry
  sin(phi)^2 : Product  OutDataType=sfix(16)  OutScaling=2^0  SaturateOnIntegerOverflow=on  InputSameDT=on  OutDataTypeStr=Inherit: Same as first input
  "Xe, m " : Outport  OutDataType=sfix(16)  OutScaling=2^0
  "Ye, m " : Outport  Port=2  OutDataType=sfix(16)  OutScaling=2^0
  "Ze, m " : Outport  Port=3  OutDataType=sfix(16)  OutScaling=2^0
  wires:
  "lat, deg"/1 -> Deg2R/1
  sin(phi)/1 -> sin(phi)^2/1, sin(phi)^2/2, Ze/1
  f/1 -> Rh/2
  Re=equatorial radius/1 -> Rh/1
  Rh/1 -> Sum2/2, Rh(1-e^2)/2
  Product1/1 -> Sum1/2
  Sum1/1 -> f/1
  const/1 -> Sum1/1
  "height, m"/1 -> Sum4/2, Sum2/1
  eccentricity^2/1(e^2) -> Product1/1, Sum3/2
  sin(phi)^2/1 -> Product1/2
  const1/1 -> Sum3/1
  Sum3/1 -> Rh(1-e^2)/1  "1-e^2"
  Rh(1-e^2)/1 -> Sum4/1
  Sum4/1 -> Ze/2
  lon,deg/1 -> Deg2R1/1
  cos(phi)/1 -> (Rh+h)cos(phi)*cos(lamb)=Xe/2, (Rh+h)cos(phi)*sin(lamb)=Ye/2
  cos(lamb)/1 -> (Rh+h)cos(phi)*cos(lamb)=Xe/3
  sin(lamb)/1 -> (Rh+h)cos(phi)*sin(lamb)=Ye/3
  Ze/1 -> "Ze, m "/1
  Deg2R/1 -> cos(phi)/1, sin(phi)/1
  Deg2R1/1 -> cos(lamb)/1, sin(lamb)/1
  Sum2/1 -> (Rh+h)cos(phi)*sin(lamb)=Ye/1, (Rh+h)cos(phi)*cos(lamb)=Xe/1
  (Rh+h)cos(phi)*cos(lamb)=Xe/1 -> "Xe, m "/1
  (Rh+h)cos(phi)*sin(lamb)=Ye/1 -> "Ye, m "/1

== system MyPCImages/Position and Attitude Filter/GPS Update/Detect Change ==
  Data : Inport  OutDataType=sfix(16)  OutScaling=2^0
  Abs1 : Abs  SampleTime=T
  Difference1 : simulink/Discrete/Difference  SystemSampleTime=-1  ICPrevInput=0.0  OutMin=[]  OutMax=[]  OutDataType=sfix(16)  OutScaling=2^-10  DoSatur=off
  Saturation1 : Saturate  UpperLimit=1  LowerLimit=0  SampleTime=T
  change? : Outport  OutDataType=sfix(16)  OutScaling=2^0
  wires:
  Saturation1/1 -> change?/1
  Data/1 -> Difference1/1
  Abs1/1 -> Saturation1/1
  Difference1/1 -> Abs1/1

== system MyPCImages/Position and Attitude Filter/GPS Update/Detect Change1 ==
  Data : Inport  OutDataType=sfix(16)  OutScaling=2^0
  Abs1 : Abs  SampleTime=T
  Difference1 : simulink/Discrete/Difference  SystemSampleTime=-1  ICPrevInput=0.0  OutMin=[]  OutMax=[]  OutDataType=sfix(16)  OutScaling=2^-10  DoSatur=off
  Saturation1 : Saturate  UpperLimit=1  LowerLimit=0  SampleTime=T
  change? : Outport  OutDataType=sfix(16)  OutScaling=2^0
  wires:
  Difference1/1 -> Abs1/1
  Abs1/1 -> Saturation1/1
  Data/1 -> Difference1/1
  Saturation1/1 -> change?/1

== system MyPCImages/Position and Attitude Filter/GPS Update/Detect Change2 ==
  Data : Inport  OutDataType=sfix(16)  OutScaling=2^0
  Abs1 : Abs  SampleTime=T
  Difference1 : simulink/Discrete/Difference  SystemSampleTime=-1  ICPrevInput=0.0  OutMin=[]  OutMax=[]  OutDataType=sfix(16)  OutScaling=2^-10  DoSatur=off
  Saturation1 : Saturate  UpperLimit=1  LowerLimit=0  SampleTime=T
  change? : Outport  OutDataType=sfix(16)  OutScaling=2^0
  wires:
  Saturation1/1 -> change?/1
  Data/1 -> Difference1/1
  Abs1/1 -> Saturation1/1
  Difference1/1 -> Abs1/1

== system MyPCImages/Position and Attitude Filter/Geod2LTP1/ECEF2LTP (UEN) ==
  ECEF coordinates : Inport  OutDataType=sfix(16)  OutScaling=2^0
  "Long, Lat" : Inport  Port=2  OutDataType=sfix(16)  OutScaling=2^0
  Deg2R : Gain  Gain=pi/180  ParameterDataType=sfix(16)  ParameterScaling=2^0  OutDataType=sfix(16)  OutScaling=2^0  SaturateOnIntegerOverflow=on  OutDataTypeStr=Inherit: Same as input  ParamDataTypeStr=Inherit: Same as input
  Demux3 : Demux  Outputs=2
  From Body to Universal1 : Subsystem
  Product1 : Product  Multiplication=Matrix(*)  OutDataType=sfix(16)  OutScaling=2^0  SaturateOnIntegerOverflow=on  InputSameDT=on  OutDataTypeStr=Inherit: Same as first input
  Out : Outport  OutDataType=sfix(16)  OutScaling=2^0
  wires:
  "Long, Lat"/1 -> Deg2R/1
  Product1/1 -> Out/1
  Demux3/2 -> From Body to Universal1/2(lat)
  Demux3/1 -> From Body to Universal1/1(long)
  Deg2R/1 -> Demux3/1
  ECEF coordinates/1 -> Product1/2
  From Body to Universal1/1(DCM) -> Product1/1
